simulink model "single_phase_multilevel"  (R2025a)
settings: Solver=ode1be  StartTime=0.0  StopTime=simlength  FixedStep=tc  RelTol=1e-3
values from neighbouring files (symbols this model uses):
  Vfc1_base = Udc/5    [plotting_results.m]    (also in plotting_results_hf.m)
  Vfc2_base = 2*Vfc1_base    [plotting_results.m]    (also in plotting_results_hf.m)
  Vfc3_base = 3*Vfc1_base    [plotting_results.m]    (also in plotting_results_hf.m)
  Vfc4_base = 4*Vfc1_base    [plotting_results.m]    (also in plotting_results_hf.m)
undefined symbols (not defined in the file or in its folder): DThs_init, g0_4Hz, g1_4Hz, I_FS, kalman_omega, kalman_theta, ki_i_inv, ki_v_inv, kp_i_inv, kp_v_inv, Lconn, LFu1, m_dead_time, m_duty_open_loop, magnitude, n1, n10, omega_ref, phase_shift_mod11, phase_shift_mod21, phase_shift_mod31, phase_shift_mod41, phase_shift_mod51, precharge_off, q1kalman, q2kalman, Rbalance, Rconn, RFu, Rg_off, Rg_on, Rkalman, RLFu1, Rprecharge, Tambient, tc, time_pwm_enable, tPWM, ts, V_FS, VCFc_5_init, Vgate_base, weigth
libraries: fl_lib x281, nesl_utility x97, ee_lib x15, simulink x1
(part 6 of 6)

== system single_phase_multilevel/output_filter/instantaneus_power/rms3 ==
  iout : Inport
  Gain : Gain  Gain=n10-1
  Gain1 : Gain  Gain=1/n10
  Math Function : Math  Operator=magnitude^2  SignedPower=on
  Sqrt : Sqrt
  Sum : Sum  Inputs=|++
  Unit Delay : UnitDelay  SampleTime=ts  HasFrameUpgradeWarning=on
  Out1 : Outport  VectorParamsAs1DForOutWhenUnconnected=off
  wires:
  Gain/1 -> Sum/2
  Sqrt/1 -> Out1/1
  Math Function/1 -> Sum/1
  Unit Delay/1 -> Gain/1
  Gain1/1 -> Unit Delay/1, Sqrt/1
  Sum/1 -> Gain1/1
  iout/1 -> Math Function/1

== system single_phase_multilevel/output_filter/voltage_measure/voltage_measure ==
  C4_100n : fl_lib/Electrical/Electrical Elements/Capacitor  c=100e-9 F  r=1e-6 Ohm  g=0 1/Ohm  i_specify=off  i_priority=None  i=0 A  i_nominal_specify=off  i_nominal_value=1  i_nominal_unit=A  v_specify=off  v_priority=None  v=0 V  v_nominal_specify=off  v_nominal_value=1  v_nominal_unit=V  vc_specify=off  vc_priority=High  vc=0 V  vc_nominal_specify=off  vc_nominal_value=1  vc_nominal_unit=V
  C5_100n : fl_lib/Electrical/Electrical Elements/Capacitor  c=100e-9 F  r=1e-6 Ohm  g=0 1/Ohm  i_specify=off  i_priority=None  i=0 A  i_nominal_specify=off  i_nominal_value=1  i_nominal_unit=A  v_specify=off  v_priority=None  v=0 V  v_nominal_specify=off  v_nominal_value=1  v_nominal_unit=V  vc_specify=off  vc_priority=High  vc=0 V  vc_nominal_specify=off  vc_nominal_value=1  vc_nominal_unit=V
  Electrical Reference{1..4} (4 alike) : fl_lib/Electrical/Electrical Elements/Electrical Reference
  PS-Simulink Converter{,1..5} (6 alike) : nesl_utility/PS-Simulink Converter  PhysicalDomain=network_engine_domain  SubClassName=ps_output  LeftPortType=input  RightPortType=output  PseudoPeriodic=off  Frequencies=[]  VectorFormat=1-D array  Unit=V  AffineConversion=off
  R10_5k : fl_lib/Electrical/Electrical Elements/Resistor  R=5e3 Ohm  i_specify=off  i_priority=None  i=0 A  i_nominal_specify=off  i_nominal_value=1  i_nominal_unit=A  v_specify=off  v_priority=None  v=0 V  v_nominal_specify=off  v_nominal_value=1  v_nominal_unit=V
  R11_10R : fl_lib/Electrical/Electrical Elements/Resistor  R=10 Ohm  i_specify=off  i_priority=None  i=0 A  i_nominal_specify=off  i_nominal_value=1  i_nominal_unit=A  v_specify=off  v_priority=None  v=0 V  v_nominal_specify=off  v_nominal_value=1  v_nominal_unit=V
  R6_12k : fl_lib/Electrical/Electrical Elements/Resistor  R=12e3 Ohm  i_specify=off  i_priority=None  i=0 A  i_nominal_specify=off  i_nominal_value=1  i_nominal_unit=A  v_specify=off  v_priority=None  v=0 V  v_nominal_specify=off  v_nominal_value=1  v_nominal_unit=V
  R7_12k : fl_lib/Electrical/Electrical Elements/Resistor  R=12e3 Ohm  i_specify=off  i_priority=None  i=0 A  i_nominal_specify=off  i_nominal_value=1  i_nominal_unit=A  v_specify=off  v_priority=None  v=0 V  v_nominal_specify=off  v_nominal_value=1  v_nominal_unit=V
  R8_5k : fl_lib/Electrical/Electrical Elements/Resistor  R=5e3 Ohm  i_specify=off  i_priority=None  i=0 A  i_nominal_specify=off  i_nominal_value=1  i_nominal_unit=A  v_specify=off  v_priority=None  v=0 V  v_nominal_specify=off  v_nominal_value=1  v_nominal_unit=V
  Voltage Sensor{,1..5} (6 alike) : fl_lib/Electrical/Electrical Sensors/Voltage Sensor
  opa-2350 : Subsystem  mask{V_opamp_pos=15, V_opamp_neg=-15, A=1e6}
      mask prompts: V_opamp_pos "V+"; V_opamp_neg "V-"; A "Open Loop Gain"
      mask help: rail to rail op-amp
      mask Help: eval('open opa2350.pdf')
      mask Display:
      | disp('OPA-2350');
      | port_label('lconn', 1, 'in(+)');
      | port_label('lconn', 2, 'in(-)');
      | port_label('rconn', 1, 'out');
  u12 : Scope  NumInputPorts=2
      settings: ActiveDisplayYMinimum=-28.07399  ActiveDisplayYMaximum=50.54623  DataLoggingVariableName=ScopeData2
  u23 : Scope  NumInputPorts=2
      settings: ActiveDisplayYMinimum=-17.37114  ActiveDisplayYMaximum=17.05862  DataLoggingVariableName=ScopeData3
  udc_m : Scope
      settings: ActiveDisplayYMinimum=-0.79008  ActiveDisplayYMaximum=0.7753
  uout_measure : Scope
      settings: ActiveDisplayYMinimum=-0.32542  ActiveDisplayYMaximum=0.31911
  u+ : PMIOPort  Side=Left
  u- : PMIOPort  Port=2  Side=Left
  wires:
  PS-Simulink Converter3/1 -> u23/1
  PS-Simulink Converter4/1 -> u23/2
  PS-Simulink Converter2/1 -> u12/2
  PS-Simulink Converter1/1 -> u12/1
  PS-Simulink Converter/1 -> uout_measure/1
  PS-Simulink Converter5/1 -> udc_m/1
  connections:
  Voltage Sensor3/RConn1 -- PS-Simulink Converter3/LConn1
  Voltage Sensor4/RConn1 -- PS-Simulink Converter4/LConn1
  Voltage Sensor4/RConn2 -- Electrical Reference4/LConn1 -- Voltage Sensor3/RConn2
  Voltage Sensor2/RConn1 -- PS-Simulink Converter2/LConn1
  Electrical Reference3/LConn1 -- Voltage Sensor2/RConn2 -- Voltage Sensor1/RConn2
  Voltage Sensor1/RConn1 -- PS-Simulink Converter1/LConn1
  PS-Simulink Converter/LConn1 -- Voltage Sensor/RConn1
  Voltage Sensor/RConn2 -- Electrical Reference1/LConn1
  Voltage Sensor/LConn1 -- C4_100n/RConn1 -- R10_5k/RConn1 -- R11_10R/RConn1
  Electrical Reference2/LConn1 -- C5_100n/RConn1 -- R8_5k/RConn1
  R6_12k/LConn1 -- C5_100n/LConn1 -- Voltage Sensor4/LConn1 -- opa-2350/LConn1 -- R8_5k/LConn1
  Voltage Sensor2/LConn1 -- u-/RConn1 -- Voltage Sensor5/RConn2 -- R7_12k/RConn1
  Voltage Sensor1/LConn1 -- u+/RConn1 -- Voltage Sensor5/LConn1 -- R6_12k/RConn1
  R10_5k/LConn1 -- R7_12k/LConn1 -- C4_100n/LConn1 -- Voltage Sensor3/LConn1 -- opa-2350/LConn2
  R11_10R/LConn1 -- opa-2350/RConn1
  Voltage Sensor5/RConn1 -- PS-Simulink Converter5/LConn1

== system single_phase_multilevel/vi_ctrl/modulator1/triangle_1 ==
  Constant : Constant  Value=pi/2
  Product : Product  Inputs=*/
  Sine Wave : Sin  Frequency=2*pi/tPWM  Phase=phase_shift_mod11  SampleTime=0
  Trigonometric Function : Trigonometry  Operator=asin
  carry_mod11 : Outport
  wires:
  Constant/1 -> Product/2
  Sine Wave/1 -> Trigonometric Function/1
  Trigonometric Function/1 -> Product/1
  Product/1 -> carry_mod11/1

== system single_phase_multilevel/vi_ctrl/modulator2/triangle_1 ==
  Constant : Constant  Value=pi/2
  Product : Product  Inputs=*/
  Sine Wave : Sin  Frequency=2*pi/tPWM  Phase=phase_shift_mod21  SampleTime=0
  Trigonometric Function : Trigonometry  Operator=asin
  carry_mod21 : Outport
  wires:
  Trigonometric Function/1 -> Product/1
  Sine Wave/1 -> Trigonometric Function/1
  Constant/1 -> Product/2
  Product/1 -> carry_mod21/1

== system single_phase_multilevel/vi_ctrl/modulator3/triangle_1 ==
  Constant : Constant  Value=pi/2
  Product : Product  Inputs=*/
  Sine Wave : Sin  Frequency=2*pi/tPWM  Phase=phase_shift_mod31  SampleTime=0
  Trigonometric Function : Trigonometry  Operator=asin
  carry_mod21 : Outport
  wires:
  Product/1 -> carry_mod21/1
  Constant/1 -> Product/2
  Sine Wave/1 -> Trigonometric Function/1
  Trigonometric Function/1 -> Product/1

== system single_phase_multilevel/vi_ctrl/modulator4/triangle_1 ==
  Constant : Constant  Value=pi/2
  Product : Product  Inputs=*/
  Sine Wave : Sin  Frequency=2*pi/tPWM  Phase=phase_shift_mod41  SampleTime=0
  Trigonometric Function : Trigonometry  Operator=asin
  carry_mod21 : Outport
  wires:
  Product/1 -> carry_mod21/1
  Constant/1 -> Product/2
  Sine Wave/1 -> Trigonometric Function/1
  Trigonometric Function/1 -> Product/1

== system single_phase_multilevel/vi_ctrl/modulator5/triangle_1 ==
  Constant : Constant  Value=pi/2
  Product : Product  Inputs=*/
  Sine Wave : Sin  Frequency=2*pi/tPWM  Phase=phase_shift_mod51  SampleTime=0
  Trigonometric Function : Trigonometry  Operator=asin
  carry_mod21 : Outport
  wires:
  Trigonometric Function/1 -> Product/1
  Sine Wave/1 -> Trigonometric Function/1
  Constant/1 -> Product/2
  Product/1 -> carry_mod21/1

== system single_phase_multilevel/vi_ctrl/single_phase_contrl_system/acquisition_and_scaling_current ==
  in : Inport
  1/Ti5 : Gain  Gain=1/I_FS  SaturateOnIntegerOverflow=on  OutDataTypeStr=Inherit: Same as input  ParamDataTypeStr=Inherit: Same as input
  Unit Delay4 : UnitDelay  SampleTime=ts  HasFrameUpgradeWarning=on
  Zero-Order Hold1 : ZeroOrderHold  SampleTime=ts
  out : Outport
  wires:
  in/1 -> Zero-Order Hold1/1
  1/Ti5/1 -> Unit Delay4/1
  Zero-Order Hold1/1 -> 1/Ti5/1
  Unit Delay4/1 -> out/1

== system single_phase_multilevel/vi_ctrl/single_phase_contrl_system/acquisition_and_scaling_voltage ==
  in : Inport
  1/Ti1 : Gain  Gain=1/V_FS  SaturateOnIntegerOverflow=on  OutDataTypeStr=Inherit: Same as input  ParamDataTypeStr=Inherit: Same as input
  Unit Delay4 : UnitDelay  SampleTime=ts  HasFrameUpgradeWarning=on
  Zero-Order Hold2 : ZeroOrderHold  SampleTime=ts
  out : Outport
  wires:
  1/Ti1/1 -> Unit Delay4/1
  Zero-Order Hold2/1 -> 1/Ti1/1
  Unit Delay4/1 -> out/1
  in/1 -> Zero-Order Hold2/1

== system single_phase_multilevel/vi_ctrl/single_phase_contrl_system/alpha_beta_transformation_i ==
  in : Inport
  Constant1 : Constant  Value=omega_ref
  Constant3 : Constant  Value=q1kalman
  Constant4 : Constant  Value=q2kalman
  Constant5 : Constant  Value=Rkalman
  Constant6 : Constant  Value=ts
  Gain : Gain  Gain=-1
  kalman_observer : MATLAB Function  TreatAsAtomicUnit=on  SystemSampleTime=ts
  alpha : Outport
  beta : Outport  Port=2
  wires:
  Constant4/1 -> kalman_observer/5(q2)
  Constant3/1 -> kalman_observer/4(q1)
  Constant5/1 -> kalman_observer/6(r)
  Constant6/1 -> kalman_observer/3(Ts)
  in/1 -> kalman_observer/1(y)
  Constant1/1 -> kalman_observer/2(w)
  kalman_observer/2(h2_hat) -> Gain/1
  kalman_observer/1(h1_hat) -> alpha/1
  Gain/1 -> beta/1

== system single_phase_multilevel/vi_ctrl/single_phase_contrl_system/alpha_beta_transformation_v ==
  in : Inport
  Constant1 : Constant  Value=omega_ref
  Constant3 : Constant  Value=q1kalman
  Constant4 : Constant  Value=q2kalman
  Constant5 : Constant  Value=Rkalman
  Constant6 : Constant  Value=ts
  Gain : Gain  Gain=-1
  kalman_observer : MATLAB Function  TreatAsAtomicUnit=on  SystemSampleTime=ts
  alpha : Outport
  beta : Outport  Port=2
  wires:
  Gain/1 -> beta/1
  kalman_observer/1(h1_hat) -> alpha/1
  kalman_observer/2(h2_hat) -> Gain/1
  Constant1/1 -> kalman_observer/2(w)
  in/1 -> kalman_observer/1(y)
  Constant6/1 -> kalman_observer/3(Ts)
  Constant5/1 -> kalman_observer/6(r)
  Constant3/1 -> kalman_observer/4(q1)
  Constant4/1 -> kalman_observer/5(q2)

== system single_phase_multilevel/vi_ctrl/single_phase_contrl_system/alphabeta2dq ==
  note: va=V cos(wt)
      | vb=V cos(wt-2pi/3)
      | vc=V cos(wt+2pi/3)
  alpha : Inport
  beta : Inport  Port=2
  wt : Inport  Port=3
  Product{,1..3} (4 alike) : Product  RndMeth=Zero
  Sum : Sum
  Sum1 : Sum  Inputs=-+
  To Workspace1 : ToWorkspace  VariableName=id_pu_modA_sim  SampleTime=ts
      settings: MaxDataPoints=Ns
  To Workspace2 : ToWorkspace  VariableName=iq_pu_modA_sim  SampleTime=ts
      settings: MaxDataPoints=Ns
  Trigonometric Function : Trigonometry  Operator=cos
  Trigonometric Function1 : Trigonometry
  "d " : Outport  VectorParamsAs1DForOutWhenUnconnected=off
  "q " : Outport  Port=2  VectorParamsAs1DForOutWhenUnconnected=off
  wires:
  wt/1 -> Trigonometric Function1/1, Trigonometric Function/1
  Trigonometric Function/1 -> [cos]
  Trigonometric Function1/1 -> [sin]
  [cos] -> Product/1
  alpha/1 -> Product/2, Product2/2
  Product/1 -> Sum/1
  Product1/1 -> Sum/2
  [sin] -> Product1/1
  beta/1 -> Product1/2, Product3/2
  Sum/1 -> To Workspace1/1, "d "/1
  [sin] -> Product2/1
  Product2/1 -> Sum1/1
  Product3/1 -> Sum1/2
  [cos] -> Product3/1
  Sum1/1 -> To Workspace2/1, "q "/1

== system single_phase_multilevel/vi_ctrl/single_phase_contrl_system/dq2alphabeta ==
  d : Inport
  q : Inport  Port=2
  wt : Inport  Port=3
  Product{,1..3} (4 alike) : Product  RndMeth=Zero
  Sum : Sum  Inputs=+-
  Sum1 : Sum
  Trigonometric Function : Trigonometry  Operator=cos
  Trigonometric Function1 : Trigonometry
  alpha : Outport  VectorParamsAs1DForOutWhenUnconnected=off
  wires:
  [cos] -> Product3/1
  Product3/1 -> Sum1/2
  Product2/1 -> Sum1/1
  [sin] -> Product2/1
  Sum/1 -> alpha/1
  q/1 -> Product3/2, Product1/2
  [sin] -> Product1/1
  Product1/1 -> Sum/2
  Product/1 -> Sum/1
  d/1 -> Product2/2, Product/2
  [cos] -> Product/1
  Trigonometric Function1/1 -> [sin]
  Trigonometric Function/1 -> [cos]
  wt/1 -> Trigonometric Function/1, Trigonometric Function1/1

== system single_phase_multilevel/vi_ctrl/single_phase_contrl_system/phase_gen ==
  load_estimator : Subsystem
  signal_generator : Subsystem
  theta : Outport
  wires:
  signal_generator/1(theta) -> theta/1

== system single_phase_multilevel/vi_ctrl/single_phase_contrl_system/pi_d ==
  id_tilde : Inport
  1/Ti : Gain  Gain=kp_i_inv  SaturateOnIntegerOverflow=on  OutDataTypeStr=Inherit: Same as input  ParamDataTypeStr=Inherit: Same as input
  Sum1 : Sum  Inputs=+++  SaturateOnIntegerOverflow=on
  Sum3 : Sum  Inputs=-+  SaturateOnIntegerOverflow=on
  To Workspace3 : ToWorkspace  VariableName=id_ctrl_out_modA_sim  SampleTime=ts
      settings: MaxDataPoints=Ns
  Unit Delay4 : UnitDelay  SampleTime=ts  HasFrameUpgradeWarning=on
  kp2 : Gain  Gain=ki_i_inv*ts  SaturateOnIntegerOverflow=on  OutDataTypeStr=Inherit: Same as input  ParamDataTypeStr=Inherit: Same as input
  ud_out_lim : Saturate  UpperLimit=1  LowerLimit=-1
  Vd_out : Outport  VectorParamsAs1DForOutWhenUnconnected=off
  wires:
  id_tilde/1 -> kp2/1, 1/Ti/1
  Sum1/1 -> ud_out_lim/1
  kp2/1 -> Sum1/2
  1/Ti/1 -> Sum1/1, Sum3/1
  Unit Delay4/1 -> Sum1/3
  Sum3/1 -> Unit Delay4/1
  ud_out_lim/1 -> To Workspace3/1, Vd_out/1, Sum3/2

== system single_phase_multilevel/vi_ctrl/single_phase_contrl_system/pi_q ==
  iq_tilde : Inport
  1/Ti : Gain  Gain=kp_i_inv  SaturateOnIntegerOverflow=on  OutDataTypeStr=Inherit: Same as input  ParamDataTypeStr=Inherit: Same as input
  Sum1 : Sum  Inputs=+++  SaturateOnIntegerOverflow=on
  Sum3 : Sum  Inputs=-+  SaturateOnIntegerOverflow=on
  To Workspace3 : ToWorkspace  VariableName=iq_ctrl_out_modA_sim  SampleTime=ts
      settings: MaxDataPoints=Ns
  Unit Delay4 : UnitDelay  SampleTime=ts  HasFrameUpgradeWarning=on
  kp2 : Gain  Gain=ki_i_inv*ts  SaturateOnIntegerOverflow=on  OutDataTypeStr=Inherit: Same as input  ParamDataTypeStr=Inherit: Same as input
  ud_out_lim : Saturate  UpperLimit=1  LowerLimit=-1
  Vd_out : Outport  VectorParamsAs1DForOutWhenUnconnected=off
  wires:
  ud_out_lim/1 -> Vd_out/1, To Workspace3/1, Sum3/2
  Sum3/1 -> Unit Delay4/1
  Unit Delay4/1 -> Sum1/3
  1/Ti/1 -> Sum3/1, Sum1/1
  kp2/1 -> Sum1/2
  Sum1/1 -> ud_out_lim/1
  iq_tilde/1 -> 1/Ti/1, kp2/1

== system single_phase_multilevel/vi_ctrl/single_phase_contrl_system/pi_v ==
  e : Inport
  1/Ti : Gain  Gain=kp_v_inv  SaturateOnIntegerOverflow=on  OutDataTypeStr=Inherit: Same as input  ParamDataTypeStr=Inherit: Same as input
  Sum1 : Sum  Inputs=+++  SaturateOnIntegerOverflow=on
  Sum3 : Sum  Inputs=-+  SaturateOnIntegerOverflow=on
  Unit Delay4 : UnitDelay  SampleTime=ts  HasFrameUpgradeWarning=on
  i_out_lim : Saturate  UpperLimit=0.869565217391304  LowerLimit=0
  kp2 : Gain  Gain=ki_v_inv*ts  SaturateOnIntegerOverflow=on  OutDataTypeStr=Inherit: Same as input  ParamDataTypeStr=Inherit: Same as input
  i_ref_internal : Outport  VectorParamsAs1DForOutWhenUnconnected=off
  tag scope: inverter_current_reference=global
  wires:
  i_out_lim/1 -> [inverter_current_reference], i_ref_internal/1, Sum3/2
  Sum3/1 -> Unit Delay4/1
  Unit Delay4/1 -> Sum1/3
  1/Ti/1 -> Sum3/1, Sum1/1
  kp2/1 -> Sum1/2
  Sum1/1 -> i_out_lim/1
  e/1 -> kp2/1, 1/Ti/1

== system single_phase_multilevel/vi_ctrl/single_phase_contrl_system/reference_flt ==
  input : Inport
  Gain3 : Gain  Gain=g1_4Hz
  Gain6 : Gain  Gain=g0_4Hz
  Sum : Sum  Inputs=|++
  Unit Delay1 : UnitDelay  SampleTime=ts  HasFrameUpgradeWarning=on
  output : Outport  VectorParamsAs1DForOutWhenUnconnected=off
  wires:
  Gain6/1 -> Sum/1
  input/1 -> Gain6/1
  Unit Delay1/1 -> Gain3/1
  Gain3/1 -> Sum/2
  Sum/1 -> Unit Delay1/1, output/1

== system single_phase_multilevel/output_filter/voltage_measure/voltage_measure/opa-2350 ==
  DC Voltage Source : fl_lib/Electrical/Electrical Sources/DC Voltage Source  v0=V_opamp_pos V
  DC Voltage Source1 : fl_lib/Electrical/Electrical Sources/DC Voltage Source  v0=V_opamp_neg V
  Diode{,1..3} (4 alike) : ee_lib/Semiconductors & Converters/Diode  ModelType=ee.enum.diode.modelType.pwl  TableType=ee.enum.diode.tableType.IfMat  IfMat=[.07, .12, .19, 1.75, 4.24, 7.32, 11.2; .16, .3, .72, 2.14, 5.02, 8.35, 13.12] A  VfMat=[.9, 1.15, 1.25, 1.5, 1.75, 2.17, 2.6, 2.85; .58, .68, .75, 1.1, 1.38, 1.77, 2.27, 2.7] V  TjVec=[25, 125] degC  VfVec=[.5, .7, .9, 1.3, 1.7, 2.1, 2.5] V  IfVec=[.1, .2, .5, 1, 2, 4, 7, 10] A  IrMat=[1e-06, 2e-06, 5e-06, 1e-05, 2.5e-05, 5e-05, .0001; 2e-06, 5e-06, 1e-05, 4e-05, 8e-05, .0002, .0005] A  VrMat=[10, 100, 200, 250, 300, 325, 350; 10, 70, 160, 220, 270, 300, 320] V  VrVec=[10, 20, 40, 50, 70, 80, 100] V  IrVec=[1e-06, 2e-06, 5e-06, 1e-05, 2e-05, 5e-05, .0001] A  Vf=0.6 V  Ron=0.3 Ohm  Goff=1e-8 S  prmExp=ee.enum.diode.expParam.useTwo  I12=[.0137, .545] A  V12=[.6, .7] V  RS=0 Ohm  Tmeas=25 degC  IS=1e-12 A  ec=1  I1=0.0137 A  V1=0.6 V  N_series=1  N_parallel=1  ZenerEnable=false  Rz=0.3 Ohm  BV=inf V  C_param=ee.enum.diode.capParam.fixed  CJ=0 pF  CJ0=5 pF  Vvec=[.1, 10, 100] V  Cvec=[3.5, 1, .4] pF  VJ=1 V  Mgrad=0.5  FC=0.5  Q_param=ee.enum.diode.recoveryParam.off  iRM=-7.15 A  iF=4 A  didt=-750 A/us  trr_factor=3  trr=115 ns  Qrr=150 nA*s  Vr=-600 V  Ls=150 nH  Erec=0.03 J  TT=50 ns  tau=100 ns  T_param=ee.enum.diode.temperatureParam.off  Tdevice=25 degC  I1_T2=0.245 A  V1_T2=0.5 V  IS_T2=1.25e-7 A  Tmeas2=125 degC  XTI_param=ee.enum.diode.xtiParam.pn  XTI=3  EG_param=ee.enum.diode.egapParam.material_si  EG=1.11 eV  dBVdT=0 V/K  enable_fault_input=simscape.enum.onoff.off  i_specify=off  i_priority=None  i=0 A  i_nominal_specify=off  i_nominal_value=1  i_nominal_unit=A  v_specify=off  v_priority=None  v=0 V  v_nominal_specify=off  v_nominal_value=1  v_nominal_unit=V  v_capacitor_specify=off  v_capacitor_priority=None  v_capacitor=0 V  v_capacitor_nominal_specify=off  v_capacitor_nominal_value=1  v_capacitor_nominal_unit=V  Qj_specify=off  Qj_priority=High  Qj=0 C  Qj_nominal_specify=off  Qj_nominal_value=1  Qj_nominal_unit=C  i_diode_specify=off  i_diode_priority=None  i_diode=0 A  i_diode_nominal_specify=off  i_diode_nominal_value=1  i_diode_nominal_unit=A  v_diode_specify=off  v_diode_priority=None  v_diode=0 V  v_diode_nominal_specify=off  v_diode_nominal_value=1  v_diode_nominal_unit=V  i_capacitor_specify=off  i_capacitor_priority=None  i_capacitor=0 A  i_capacitor_nominal_specify=off  i_capacitor_nominal_value=1  i_capacitor_nominal_unit=A  power_dissipated_specify=off  power_dissipated_priority=None  power_dissipated=0 W  power_dissipated_nominal_specify=off  power_dissipated_nominal_value=1  power_dissipated_nominal_unit=W  fidelity_level=ee.enum.diode.fidelity.includeChargeDyn  rec_loss_model=ee.enum.diode.reverseRecoveryModel.fixed  ErecVal=0 J  scaleWithIandV=true  ErecMat=zeros(2, 3) J  TjrecVec=[298.15, 398.15] K  IfrecVec=[.1, 1, 10] A  IrecVal=10 A  VrecVal=10 V  tFilter=1 / 1000 / 100 s  thermal_network_parameterization=ee.enum.thermalNetworkTopology.junctionCase  Rth=[0, 10] K/W  Rth_Cauer=[1, 3, 10] K/W  Rth_Foster=[4, 6] K/W  thermal_mass_parameterization=ee.enum.thermalNetwork.timeconstant  thermal_mass=[0, 1] J/K  thermal_mass_Cauer=[.1, .3, 1] J/K  thermal_mass_Foster=[1.5, 3] J/K  thermal_time_constant=[0, 10] s  thermal_time_constant_Cauer=[1, 3, 10] s  thermal_time_constant_Foster=[6, 18] s  thermal_mass_initial_temperatures=[25, 25] degC  thermal_mass_initial_temperatures_Cauer=[25, 25, 25] degC  junction_thermal_mass=0.01 J/K  Tvec_initial_Foster=[25, 25, 25, 25] degC  no_thermal_network=0  junction_temperature_specify=off  junction_temperature_priority=None  junction_temperature=25 degC  junction_temperature_nominal_specify=off  junction_temperature_nominal_value=1  junction_temperature_nominal_unit=degC
  Electrical Reference5 : fl_lib/Electrical/Electrical Elements/Electrical Reference
  Electrical Reference6 : fl_lib/Electrical/Electrical Elements/Electrical Reference
  Finite-Gain Op-Amp : ee_lib/Integrated Circuits/Finite-Gain Op-Amp  A=A  Rin=1e6 Ohm  Rout=100 Ohm  Vmin=V_opamp_neg V  Vmax=V_opamp_pos V  noise_mode=ee.enum.mode.disabled  v_noise=30e-9 V/Hz^(1/2)  noise_prm=ee.enum.ic.noiseParameterization.same  i_noise=0.5e-12 A/Hz^(1/2)  ip_noise=0.5e-12 A/Hz^(1/2)  in_noise=0.5e-12 A/Hz^(1/2)  sample_time=1e-3 s  repeatability=ee.enum.ic.repeatability.notRepeatable  auto_seed_v=1196140742  auto_seed_ip=2348838240  auto_seed_in=4112460543  user_seed_v=0  user_seed_ip=0  user_seed_in=0
      settings: InternalSimscapePortConfiguration="{\"Bottom\":[],\"Left\":[{\"id\":\"p\",\"label\":\"+\",\"type\":\"foundation.electrical.electrical\"},{\"id\":\"n\",\"label\":\"-\",\"type\":\"foundation.electrical.electrical\"}],\"Right\":[{\"id\":\"out\",\"label\":\"\",\"type\":\"foundation.electrical.electrical\"}],\"Top\":[]}"
  in(+) : PMIOPort  Side=Left
  out : PMIOPort  Port=2  Side=Right
  in(-) : PMIOPort  Port=3  Side=Left
  connections:
  Finite-Gain Op-Amp/LConn1 -- in(+)/RConn1 -- Diode1/RConn1 -- Diode/LConn1
  Diode/RConn1 -- DC Voltage Source/LConn1 -- Diode2/RConn1
  out/RConn1 -- Finite-Gain Op-Amp/RConn1
  Diode3/RConn1 -- Diode2/LConn1 -- in(-)/RConn1 -- Finite-Gain Op-Amp/LConn2
  Diode1/LConn1 -- DC Voltage Source1/LConn1 -- Diode3/LConn1
  Electrical Reference6/LConn1 -- DC Voltage Source1/RConn1
  Electrical Reference5/LConn1 -- DC Voltage Source/RConn1

== system single_phase_multilevel/vi_ctrl/single_phase_contrl_system/phase_gen/load_estimator ==
  theta : Inport
  Gain : Gain  Gain=kalman_omega
  Gain1 : Gain  Gain=kalman_theta
  Gain5 : Gain  Gain=ts
  Sum : Sum  Inputs=-+|
  Sum1 : Sum  Inputs=|++
  Sum2 : Sum  Inputs=|++
  Sum8 : Sum  Inputs=++|
  Unit Delay1 : UnitDelay  SampleTime=ts  HasFrameUpgradeWarning=on
  Unit Delay2 : UnitDelay  SampleTime=ts  HasFrameUpgradeWarning=on
  bounder1 : MATLAB Function  TreatAsAtomicUnit=on  SystemSampleTime=ts
  bounder2 : MATLAB Function  TreatAsAtomicUnit=on  SystemSampleTime=ts
  theta_hat : Outport  VectorParamsAs1DForOutWhenUnconnected=off
  wires:
  theta/1 -> Sum/2  "theta"
  Sum8/1 -> bounder2/1(u)
  Sum1/1 -> Unit Delay2/1
  Unit Delay2/1 -> Sum1/2, Gain5/1
  Sum2/1 -> Sum8/2
  bounder2/1(y) -> Unit Delay1/1
  bounder1/1(y) -> Gain/1, Gain1/1
  Sum/1 -> bounder1/1(u)
  Unit Delay1/1 -> Sum2/2, theta_hat/1, Sum/1  "theta_hat"
  Gain5/1 -> Sum8/1
  Gain1/1 -> Sum2/1
  Gain/1 -> Sum1/1

== system single_phase_multilevel/vi_ctrl/single_phase_contrl_system/phase_gen/signal_generator ==
  Unit Delay2 : UnitDelay  SampleTime=ts  HasFrameUpgradeWarning=on
  signal_generator : Subsystem
  theta : Outport
  wires:
  Unit Delay2/1 -> theta/1
  signal_generator/1(theta) -> Unit Delay2/1

== system single_phase_multilevel/vi_ctrl/single_phase_contrl_system/phase_gen/signal_generator/signal_generator ==
  Constant4 : Constant  Value=omega_ref
  Constant7 : Constant
  Product2 : Product  RndMeth=Zero
  Sum4 : Sum  SaturateOnIntegerOverflow=on
  Unit Delay1 : UnitDelay  SampleTime=ts  HasFrameUpgradeWarning=on
  bounder : MATLAB Function  TreatAsAtomicUnit=on  SystemSampleTime=ts
  kp2 : Gain  Gain=ts  SaturateOnIntegerOverflow=on  OutDataTypeStr=Inherit: Same as input  ParamDataTypeStr=Inherit: Same as input
  theta : Outport
  wires:
  Product2/1 -> kp2/1
  bounder/1(y) -> Unit Delay1/1, theta/1
  kp2/1 -> Sum4/1
  Constant7/1 -> Product2/1
  Constant4/1 -> Product2/2
  Unit Delay1/1 -> Sum4/2
  Sum4/1 -> bounder/1(u)

== matlab function single_phase_multilevel/vi_ctrl/single_phase_contrl_system/alpha_beta_transformation_v/kalman_observer ==
  data: y input; h1_hat output; w input; Ts input; q1 input; q2 input; r input; h2_hat output
function [h1_hat, h2_hat]   = KFO(y,w,Ts,q1,q2,r)

    persistent   x1_po x2_po p11_po p12_po p21_po p22_po

    if isempty(x1_po)
        x1_po = 0;
        x2_po = 0;
        p11_po = 0;
        p12_po = 0;
        p21_po = 0;
        p22_po = 0;        
    end
    
    a11 = cos(w*Ts);
    a12 = sin(w*Ts);
    a21 = -sin(w*Ts);
    a22 = cos(w*Ts);
    
    x1_pr = a11*x1_po + a12*x2_po;
    x2_pr = a21*x1_po + a22*x2_po;
    
    p11_pr = q1 + a11*(a11*p11_po+a12*p21_po) + a12*(a11*p12_po+a12*p22_po);
    p12_pr = a21*(a11*p11_po+a12*p21_po) + a22*(a11*p12_po+a12*p22_po);
    p21_pr = a11*(a21*p11_po+a22*p21_po) + a12*(a21*p12_po+a22*p22_po);
    p22_pr = q2 + a21*(a21*p11_po+a22*p21_po) + a22*(a21*p12_po+a22*p22_po);
    
    l1 = p11_pr/(p11_pr + r);
    l2 = p21_pr/(p11_pr + r);
    
    x1_po = x1_pr + l1*(y-x1_pr);
    x2_po = x2_pr + l2*(y-x1_pr);
    
    p11_po = (1-l1)*p11_pr;
    p12_po = (1-l1)*p12_pr;
    p21_po = p21_pr-l2*p11_pr;
    p22_po = p22_pr-l2*p12_pr;
    
    h1_hat = x1_pr;
    h2_hat = x2_pr;
end

== matlab function single_phase_multilevel/vi_ctrl/single_phase_contrl_system/phase_gen/signal_generator/signal_generator/bounder ==
  data: u input; y output
function y = bounder(u)
    
    y = -pi + mod(u+3*pi,2*pi);
   
end

== matlab function single_phase_multilevel/vi_ctrl/single_phase_contrl_system/phase_gen/load_estimator/bounder1 ==
  data: u input; y output
function y = bounder(u)
    
    u = -pi + mod(u+3*pi,2*pi);
    
    y = u;
end

== matlab function single_phase_multilevel/vi_ctrl/single_phase_contrl_system/phase_gen/load_estimator/bounder2 ==
  data: u input; y output
function y = bounder(u)
    
    u = -pi + mod(u+3*pi,2*pi);
    
    y = u;
end

== matlab function single_phase_multilevel/vi_ctrl/single_phase_contrl_system/alpha_beta_transformation_i/kalman_observer ==
  data: y input; h1_hat output; w input; Ts input; q1 input; q2 input; r input; h2_hat output
function [h1_hat, h2_hat]   = KFO(y,w,Ts,q1,q2,r)

    persistent   x1_po x2_po p11_po p12_po p21_po p22_po

    if isempty(x1_po)
        x1_po = 0;
        x2_po = 0;
        p11_po = 0;
        p12_po = 0;
        p21_po = 0;
        p22_po = 0;        
    end
    
    a11 = cos(w*Ts);
    a12 = sin(w*Ts);
    a21 = -sin(w*Ts);
    a22 = cos(w*Ts);
    
    x1_pr = a11*x1_po + a12*x2_po;
    x2_pr = a21*x1_po + a22*x2_po;
    
    p11_pr = q1 + a11*(a11*p11_po+a12*p21_po) + a12*(a11*p12_po+a12*p22_po);
    p12_pr = a21*(a11*p11_po+a12*p21_po) + a22*(a11*p12_po+a12*p22_po);
    p21_pr = a11*(a21*p11_po+a22*p21_po) + a12*(a21*p12_po+a22*p22_po);
    p22_pr = q2 + a21*(a21*p11_po+a22*p21_po) + a22*(a21*p12_po+a22*p22_po);
    
    l1 = p11_pr/(p11_pr + r);
    l2 = p21_pr/(p11_pr + r);
    
    x1_po = x1_pr + l1*(y-x1_pr);
    x2_po = x2_pr + l2*(y-x1_pr);
    
    p11_po = (1-l1)*p11_pr;
    p12_po = (1-l1)*p12_pr;
    p21_po = p21_pr-l2*p11_pr;
    p22_po = p22_pr-l2*p12_pr;
    
    h1_hat = x1_pr;
    h2_hat = x2_pr;
end
